simulink model "While_ejemplo"  (Simulink 7.1)
settings: Solver=ode45  StartTime=0.0  StopTime=10.0  RelTol=1e-3
libraries: simulink x1
settings Model: Creator=Usuario  LastModifiedBy=Usuario

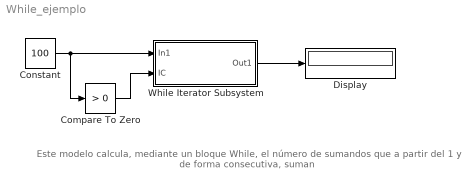
== system While_ejemplo ==
  note: Este modelo calcula, mediante un bloque While, el número de sumandos que a partir del 1 y de forma consecutiva, suman
  Compare To Zero : simulink/Logic and Bit Operations/Compare To Zero  SystemSampleTime=-1  relop=>  LogicOutDataTypeMode=uint8  ZeroCross=off
  Constant : Constant  Value=100  OutDataType=sfix(16)  OutScaling=2^0
  Display : Display
  While Iterator Subsystem : Subsystem  TreatAsAtomicUnit=on
  wires:
  Constant/1 -> While Iterator Subsystem/1(In1), Compare To Zero/1
  Compare To Zero/1 -> While Iterator Subsystem/2(IC)
  While Iterator Subsystem/1(Out1) -> Display/1

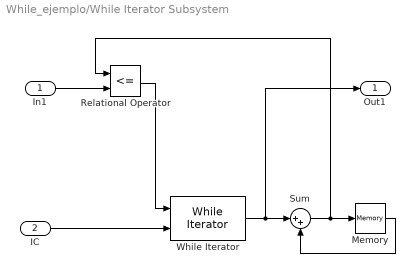
== system While_ejemplo/While Iterator Subsystem ==
  In1 : Inport  OutDataType=sfix(16)  OutScaling=2^0
  IC : Inport  Port=2  OutDataType=sfix(16)  OutScaling=2^0
  Memory : Memory  InheritSampleTime=on
  Relational Operator : RelationalOperator  Operator=<=  LogicOutDataTypeMode=boolean  OutDataTypeStr=boolean
  Sum : Sum  Inputs=|++  OutDataType=sfix(16)  OutScaling=2^0
  While Iterator : WhileIterator  MaxIters=20  ResetStates=reset  ShowIterationPort=on
  Out1 : Outport  OutDataType=sfix(16)  OutScaling=2^0
  wires:
  IC/1 -> While Iterator/2
  Relational Operator/1 -> While Iterator/1
  While Iterator/1 -> Out1/1, Sum/1
  Sum/1 -> Memory/1, Relational Operator/1
  Memory/1 -> Sum/2
  In1/1 -> Relational Operator/2
